simulink model "integrator_12B_with_contracts_Req_TUI003v1_PP"  (R2019b)
settings: Solver=FixedStepDiscrete  StartTime=0.0  StopTime=10.0  FixedStep=1.000000  RelTol=1e-3  EnableMultiTasking=on
model workspace (MAT data in the model file):
  ContractValidatorBlocksMap = containers.Map
  ContractValidatorBlocksMap.serialization.keys = {'integrator_12B/contract/validator', 'integrator_12B_with_contracts/integrator_12B_Tustin_IntegratorSpec/validator', 'integrator_12B_with_contracts_Req_TUI003v1/integrator_12B_Tustin_IntegratorSpec/validator', 'integrator_12B_with_contracts_Req_TUI003v1_PP/integrator_12B_Tustin_IntegratorSpec/validator'}
  ContractValidatorBlocksMap.serialization.values{1}.block = 'integrator_12B/contract/validator'
  ContractValidatorBlocksMap.serialization.values{1}.assumePorts = 0
  ContractValidatorBlocksMap.serialization.values{1}.guaranteePorts = 3
  ContractValidatorBlocksMap.serialization.values{1}.modeBlocksPorts = 0
  ContractValidatorBlocksMap.serialization.values{1}.portHandles.Inport = [741.001708984 742.001708984 743.001708984]
  ContractValidatorBlocksMap.serialization.values{1}.portHandles.Outport = 744.001708984
  ContractValidatorBlocksMap.serialization.values{1}.portHandles.Enable = []
  ContractValidatorBlocksMap.serialization.values{1}.portHandles.Trigger = []
  ContractValidatorBlocksMap.serialization.values{1}.portHandles.State = []
  ContractValidatorBlocksMap.serialization.values{1}.portHandles.LConn = []
  ContractValidatorBlocksMap.serialization.values{1}.portHandles.RConn = []
  ContractValidatorBlocksMap.serialization.values{1}.portHandles.Ifaction = []
  ContractValidatorBlocksMap.serialization.values{1}.portHandles.Reset = []
  ContractValidatorBlocksMap.serialization.values{1}.portConnectivity(1).Type = '1'
  ContractValidatorBlocksMap.serialization.values{1}.portConnectivity(1).Position = [365 -95]
  ContractValidatorBlocksMap.serialization.values{1}.portConnectivity(1).SrcBlock = 540.001953125
  ContractValidatorBlocksMap.serialization.values{1}.portConnectivity(1).SrcPort = 0
  ContractValidatorBlocksMap.serialization.values{1}.portConnectivity(1).DstBlock = []
  ContractValidatorBlocksMap.serialization.values{1}.portConnectivity(1).DstPort = []
  ContractValidatorBlocksMap.serialization.values{1}.portConnectivity(2).Type = '2'
  ContractValidatorBlocksMap.serialization.values{1}.portConnectivity(2).Position = [365 75]
  ContractValidatorBlocksMap.serialization.values{1}.portConnectivity(2).SrcBlock = 544.001953125
  ContractValidatorBlocksMap.serialization.values{1}.portConnectivity(2).SrcPort = 0
  ContractValidatorBlocksMap.serialization.values{1}.portConnectivity(2).DstBlock = []
  ContractValidatorBlocksMap.serialization.values{1}.portConnectivity(2).DstPort = []
  ContractValidatorBlocksMap.serialization.values{1}.portConnectivity(3).Type = '3'
  ContractValidatorBlocksMap.serialization.values{1}.portConnectivity(3).Position = [365 245]
  ContractValidatorBlocksMap.serialization.values{1}.portConnectivity(3).SrcBlock = 548.001953125
  ContractValidatorBlocksMap.serialization.values{1}.portConnectivity(3).SrcPort = 0
  ContractValidatorBlocksMap.serialization.values{1}.portConnectivity(3).DstBlock = []
  ContractValidatorBlocksMap.serialization.values{1}.portConnectivity(3).DstPort = []
  ContractValidatorBlocksMap.serialization.values{1}.portConnectivity(4).Type = '1'
  ContractValidatorBlocksMap.serialization.values{1}.portConnectivity(4).Position = [500 75]
  ContractValidatorBlocksMap.serialization.values{1}.portConnectivity(4).SrcBlock = []
  ContractValidatorBlocksMap.serialization.values{1}.portConnectivity(4).SrcPort = []
  ContractValidatorBlocksMap.serialization.values{1}.portConnectivity(4).DstBlock = 591.001708984
  ContractValidatorBlocksMap.serialization.values{1}.portConnectivity(4).DstPort = 0
  ContractValidatorBlocksMap.serialization.values{2}.block = 'integrator_12B_with_contracts/integrator_12B_Tustin_IntegratorSpec/validator'
  ContractValidatorBlocksMap.serialization.values{2}.assumePorts = 1
  ContractValidatorBlocksMap.serialization.values{2}.guaranteePorts = 1
  ContractValidatorBlocksMap.serialization.values{2}.modeBlocksPorts = 0
  ContractValidatorBlocksMap.serialization.values{2}.portHandles.Inport = [975.177368164 977.177368164]
  ContractValidatorBlocksMap.serialization.values{2}.portHandles.Outport = 1002.17736816
  ContractValidatorBlocksMap.serialization.values{2}.portHandles.Enable = []
  ContractValidatorBlocksMap.serialization.values{2}.portHandles.Trigger = []
  ContractValidatorBlocksMap.serialization.values{2}.portHandles.State = []
  ContractValidatorBlocksMap.serialization.values{2}.portHandles.LConn = []
  ContractValidatorBlocksMap.serialization.values{2}.portHandles.RConn = []
  ContractValidatorBlocksMap.serialization.values{2}.portHandles.Ifaction = []
  ContractValidatorBlocksMap.serialization.values{2}.portHandles.Reset = []
  ContractValidatorBlocksMap.serialization.values{2}.portConnectivity(1).Type = '1'
  ContractValidatorBlocksMap.serialization.values{2}.portConnectivity(1).Position = [1440 910]
  ContractValidatorBlocksMap.serialization.values{2}.portConnectivity(1).SrcBlock = 715.177368164
  ContractValidatorBlocksMap.serialization.values{2}.portConnectivity(1).SrcPort = 0
  ContractValidatorBlocksMap.serialization.values{2}.portConnectivity(1).DstBlock = []
  ContractValidatorBlocksMap.serialization.values{2}.portConnectivity(1).DstPort = []
  ContractValidatorBlocksMap.serialization.values{2}.portConnectivity(2).Type = '2'
  ContractValidatorBlocksMap.serialization.values{2}.portConnectivity(2).Position = [1440 960]
  ContractValidatorBlocksMap.serialization.values{2}.portConnectivity(2).SrcBlock = 723.177368164
  ContractValidatorBlocksMap.serialization.values{2}.portConnectivity(2).SrcPort = 0
  ContractValidatorBlocksMap.serialization.values{2}.portConnectivity(2).DstBlock = []
  ContractValidatorBlocksMap.serialization.values{2}.portConnectivity(2).DstPort = []
  ContractValidatorBlocksMap.serialization.values{2}.portConnectivity(3).Type = '1'
  ContractValidatorBlocksMap.serialization.values{2}.portConnectivity(3).Position = [1480 935]
  ContractValidatorBlocksMap.serialization.values{2}.portConnectivity(3).SrcBlock = []
  ContractValidatorBlocksMap.serialization.values{2}.portConnectivity(3).SrcPort = []
  ContractValidatorBlocksMap.serialization.values{2}.portConnectivity(3).DstBlock = 780.177368164
  ContractValidatorBlocksMap.serialization.values{2}.portConnectivity(3).DstPort = 0
  ContractValidatorBlocksMap.serialization.values{3}.block = 'integrator_12B_with_contracts_Req_TUI003v1/integrator_12B_Tustin_IntegratorSpec/validator'
  ContractValidatorBlocksMap.serialization.values{3}.assumePorts = 1
  ContractValidatorBlocksMap.serialization.values{3}.guaranteePorts = 1
  ContractValidatorBlocksMap.serialization.values{3}.modeBlocksPorts = 0
  ContractValidatorBlocksMap.serialization.values{3}.portHandles.Inport = [223.123657227 224.125366211]
  ContractValidatorBlocksMap.serialization.values{3}.portHandles.Outport = 225.12890625
  ContractValidatorBlocksMap.serialization.values{3}.portHandles.Enable = []
  ContractValidatorBlocksMap.serialization.values{3}.portHandles.Trigger = []
  ContractValidatorBlocksMap.serialization.values{3}.portHandles.State = []
  ContractValidatorBlocksMap.serialization.values{3}.portHandles.LConn = []
  ContractValidatorBlocksMap.serialization.values{3}.portHandles.RConn = []
  ContractValidatorBlocksMap.serialization.values{3}.portHandles.Ifaction = []
  ContractValidatorBlocksMap.serialization.values{3}.portHandles.Reset = []
  ContractValidatorBlocksMap.serialization.values{3}.portConnectivity(1).Type = '1'
  ContractValidatorBlocksMap.serialization.values{3}.portConnectivity(1).Position = [1440 910]
  ContractValidatorBlocksMap.serialization.values{3}.portConnectivity(1).SrcBlock = 127.121582031
  ContractValidatorBlocksMap.serialization.values{3}.portConnectivity(1).SrcPort = 0
  ContractValidatorBlocksMap.serialization.values{3}.portConnectivity(1).DstBlock = []
  ContractValidatorBlocksMap.serialization.values{3}.portConnectivity(1).DstPort = []
  ContractValidatorBlocksMap.serialization.values{3}.portConnectivity(2).Type = '2'
  ContractValidatorBlocksMap.serialization.values{3}.portConnectivity(2).Position = [1440 960]
  ContractValidatorBlocksMap.serialization.values{3}.portConnectivity(2).SrcBlock = 121.124511719
  ContractValidatorBlocksMap.serialization.values{3}.portConnectivity(2).SrcPort = 0
  ContractValidatorBlocksMap.serialization.values{3}.portConnectivity(2).DstBlock = []
  ContractValidatorBlocksMap.serialization.values{3}.portConnectivity(2).DstPort = []
  ContractValidatorBlocksMap.serialization.values{3}.portConnectivity(3).Type = '1'
  ContractValidatorBlocksMap.serialization.values{3}.portConnectivity(3).Position = [1480 935]
  ContractValidatorBlocksMap.serialization.values{3}.portConnectivity(3).SrcBlock = []
  ContractValidatorBlocksMap.serialization.values{3}.portConnectivity(3).SrcPort = []
  ContractValidatorBlocksMap.serialization.values{3}.portConnectivity(3).DstBlock = 149.117919922
  ContractValidatorBlocksMap.serialization.values{3}.portConnectivity(3).DstPort = 0
  ContractValidatorBlocksMap.serialization.values{4}.block = 'integrator_12B_with_contracts_Req_TUI003v1_PP/integrator_12B_Tustin_IntegratorSpec/validator'
  ContractValidatorBlocksMap.serialization.values{4}.assumePorts = 1
  ContractValidatorBlocksMap.serialization.values{4}.guaranteePorts = 1
  ContractValidatorBlocksMap.serialization.values{4}.modeBlocksPorts = 0
  ContractValidatorBlocksMap.serialization.values{4}.portHandles.Inport = [232.125976562 233.154296875]
  ContractValidatorBlocksMap.serialization.values{4}.portHandles.Outport = 234.124511719
  ContractValidatorBlocksMap.serialization.values{4}.portHandles.Enable = []
  ContractValidatorBlocksMap.serialization.values{4}.portHandles.Trigger = []
  ContractValidatorBlocksMap.serialization.values{4}.portHandles.State = []
  ContractValidatorBlocksMap.serialization.values{4}.portHandles.LConn = []
  ContractValidatorBlocksMap.serialization.values{4}.portHandles.RConn = []
  ContractValidatorBlocksMap.serialization.values{4}.portHandles.Ifaction = []
  ContractValidatorBlocksMap.serialization.values{4}.portHandles.Reset = []
  ContractValidatorBlocksMap.serialization.values{4}.portConnectivity(1).Type = '1'
  ContractValidatorBlocksMap.serialization.values{4}.portConnectivity(1).Position = [1440 910]
  ContractValidatorBlocksMap.serialization.values{4}.portConnectivity(1).SrcBlock = 127.121704102
  ContractValidatorBlocksMap.serialization.values{4}.portConnectivity(1).SrcPort = 0
  ContractValidatorBlocksMap.serialization.values{4}.portConnectivity(1).DstBlock = []
  ContractValidatorBlocksMap.serialization.values{4}.portConnectivity(1).DstPort = []
  ContractValidatorBlocksMap.serialization.values{4}.portConnectivity(2).Type = '2'
  ContractValidatorBlocksMap.serialization.values{4}.portConnectivity(2).Position = [1440 960]
  ContractValidatorBlocksMap.serialization.values{4}.portConnectivity(2).SrcBlock = 121.124633789
  ContractValidatorBlocksMap.serialization.values{4}.portConnectivity(2).SrcPort = 0
  ContractValidatorBlocksMap.serialization.values{4}.portConnectivity(2).DstBlock = []
  ContractValidatorBlocksMap.serialization.values{4}.portConnectivity(2).DstPort = []
  ContractValidatorBlocksMap.serialization.values{4}.portConnectivity(3).Type = '1'
  ContractValidatorBlocksMap.serialization.values{4}.portConnectivity(3).Position = [1480 935]
  ContractValidatorBlocksMap.serialization.values{4}.portConnectivity(3).SrcBlock = []
  ContractValidatorBlocksMap.serialization.values{4}.portConnectivity(3).SrcPort = []
  ContractValidatorBlocksMap.serialization.values{4}.portConnectivity(3).DstBlock = 158.119506836
  ContractValidatorBlocksMap.serialization.values{4}.portConnectivity(3).DstPort = 0
  ContractValidatorBlocksMap.serialization.uniformity = 0
  ContractValidatorBlocksMap.serialization.keyType = 'char'
  ContractValidatorBlocksMap.serialization.valueType = 'any'
  already_pp = 1
  compositionalMap.analysisNames{1} = 'integrator_12B_with_contracts_Req_TUI003v1_PP/Tustin
    | Integrator
    | (Limited, Resettable, States)'
  compositionalMap.compositionalOptions = {{''}}
  compositionalMap.selectedOptions = 1
  maskControlsMap = containers.Map
  maskControlsMap.serialization.keys = {'integrator_12B_with_contracts_Req_TUI003v1_PP/integrator_12B_Tustin_IntegratorSpec/TUI003v1'}
  maskControlsMap.serialization.values = {{'Display_counter_example_as_signals', 'Display_counter_example_as_tables', 'Display_counter_example_as_HTML_tables', 'Generate_an_outer_model_for_the_counter_example', 'Generate_an_inner_model_for_the_counter_example'}}
  maskControlsMap.serialization.uniformity = 0
  maskControlsMap.serialization.keyType = 'char'
  maskControlsMap.serialization.valueType = 'any'
  nodeNameToBlockNameMap = containers.Map
  nodeNameToBlockNameMap.serialization.keys = {'A_1', 'A_equal__equal__gt_B_1', 'Arrow_xxTustin_IntegratorSpec_7_ni_1_1', 'BL_1', 'BLc_1', 'B_1', 'Gain_1', 'In1_1', 'Logical_newline_Operator1_1', 'Logical_newline_Operator_1', 'LowerRelop1_1', 'PRE_xxTustin_IntegratorSpec_11_1', 'PRE_xxTustin_IntegratorSpec_9_1', 'Product_1', 'RelationalOperator_1', 'Saturation_newline_Dynamic_1', 'Saturation_newline_Dynamic_22_119', 'Sum1_1', 'Sum_1', 'Switch1_1', 'Switch2_1', 'Switch_1', 'TL_1', 'TLc_1', 'TUI003v1_1', 'TUI003v1_121_125', 'T_1', 'Tustin_IntegratorSpec_BL_1', 'Tustin_IntegratorSpec_IC_1', 'Tustin_IntegratorSpec_RESET_1', 'Tustin_IntegratorSpec_TL_1', 'Tustin_IntegratorSpec_T_1', 'Tustin_IntegratorSpec_xin_1', 'Tustin_IntegratorSpec_yout_1', 'Tustin_newline_Integrator_newline__lpar_Limited_comma_Resettable_comma_States_rpar__1', 'Tustin_newline_Integrator_newline__lpar_Limited_comma_Resettable_comma_States_rpar__9_120', 'UnitDelay1_1', 'UnitDelay_1', 'UpperRelop_1', 'assume_1', 'assume_127_122', 'bounds_1', 'bounds_2', 'bounds_63_125', 'branch_8_IF_1', 'branch_9_IF_1', 'guarantee_1', 'ic_1', 'integrator_12B_Tustin_IntegratorSpec_110_125', 'integrator_12B_with_contracts_Req_TUI003v1_PP', 'lo_1', 'normal_yout_operator_1', 'normalv1_operator_1', 'reset_1', 'spec137_operator_1', 'spec160_operator_1', 'spec160_operator_136_119', 'u_1', 'up_1', 'valid_1', 'xin_1', 'xxTustin_IntegratorSpec_13_operator_1', 'xxTustin_IntegratorSpec_14_operator_1', 'xxTustin_IntegratorSpec_15_operator_1', 'xxTustin_IntegratorSpec_16_operator_1', 'xxTustin_IntegratorSpec_1_operator_1', 'xxTustin_IntegratorSpec_4_operator_1', 'xxTustin_IntegratorSpec_5_operator_1', 'xxTustin_IntegratorSpec_5_rhs_2_1', 'xxTustin_IntegratorSpec_6_operator_1', 'xxTustin_IntegratorSpec_7_ni_1_init_1', 'xxTustin_IntegratorSpec_8_rhs_1', 'y_1', 'yout_1'}
  nodeNameToBlockNameMap.serialization.values{1} = 'integrator_12B_with_contracts_Req_TUI003v1_PP/integrator_12B_Tustin_IntegratorSpec/spec160_operator/A'
  nodeNameToBlockNameMap.serialization.values{2} = 'integrator_12B_with_contracts_Req_TUI003v1_PP/integrator_12B_Tustin_IntegratorSpec/spec160_operator/A ==> B'
  nodeNameToBlockNameMap.serialization.values{3} = 'integrator_12B_with_contracts_Req_TUI003v1_PP/integrator_12B_Tustin_IntegratorSpec/Arrow_xxTustin_IntegratorSpec_7_ni_1'
  nodeNameToBlockNameMap.serialization.values{4} = 'integrator_12B_with_contracts_Req_TUI003v1_PP/BL'
  nodeNameToBlockNameMap.serialization.values{5} = 'integrator_12B_with_contracts_Req_TUI003v1_PP/Tustin
    | Integrator
    | (Limited, Resettable, States)/bounds/BLc'
  nodeNameToBlockNameMap.serialization.values{6} = 'integrator_12B_with_contracts_Req_TUI003v1_PP/integrator_12B_Tustin_IntegratorSpec/spec160_operator/B'
  nodeNameToBlockNameMap.serialization.values{7} = 'integrator_12B_with_contracts_Req_TUI003v1_PP/Tustin
    | Integrator
    | (Limited, Resettable, States)/Gain'
  nodeNameToBlockNameMap.serialization.values{8} = 'integrator_12B_with_contracts_Req_TUI003v1_PP/integrator_12B_Tustin_IntegratorSpec/assume/In1'
  nodeNameToBlockNameMap.serialization.values{9} = 'integrator_12B_with_contracts_Req_TUI003v1_PP/integrator_12B_Tustin_IntegratorSpec/spec160_operator/Logical
    | Operator1'
  nodeNameToBlockNameMap.serialization.values{10} = 'integrator_12B_with_contracts_Req_TUI003v1_PP/integrator_12B_Tustin_IntegratorSpec/spec160_operator/Logical
    | Operator'
  nodeNameToBlockNameMap.serialization.values{11} = 'integrator_12B_with_contracts_Req_TUI003v1_PP/Tustin
    | Integrator
    | (Limited, Resettable, States)/Saturation
    | Dynamic/LowerRelop1'
  nodeNameToBlockNameMap.serialization.values{12} = 'integrator_12B_with_contracts_Req_TUI003v1_PP/integrator_12B_Tustin_IntegratorSpec/PRE_xxTustin_IntegratorSpec_11'
  nodeNameToBlockNameMap.serialization.values{13} = 'integrator_12B_with_contracts_Req_TUI003v1_PP/integrator_12B_Tustin_IntegratorSpec/PRE_xxTustin_IntegratorSpec_9'
  nodeNameToBlockNameMap.serialization.values{14} = 'integrator_12B_with_contracts_Req_TUI003v1_PP/Tustin
    | Integrator
    | (Limited, Resettable, States)/Product'
  nodeNameToBlockNameMap.serialization.values{15} = 'integrator_12B_with_contracts_Req_TUI003v1_PP/Tustin
    | Integrator
    | (Limited, Resettable, States)/bounds/Relational Operator'
  nodeNameToBlockNameMap.serialization.values{16} = 'integrator_12B_with_contracts_Req_TUI003v1_PP/Tustin
    | Integrator
    | (Limited, Resettable, States)/Saturation
    | Dynamic'
  nodeNameToBlockNameMap.serialization.values{17} = 'integrator_12B_with_contracts_Req_TUI003v1_PP/Tustin
    | Integrator
    | (Limited, Resettable, States)/Saturation
    | Dynamic'
  nodeNameToBlockNameMap.serialization.values{18} = 'integrator_12B_with_contracts_Req_TUI003v1_PP/Tustin
    | Integrator
    | (Limited, Resettable, States)/Sum1'
  nodeNameToBlockNameMap.serialization.values{19} = 'integrator_12B_with_contracts_Req_TUI003v1_PP/Tustin
    | Integrator
    | (Limited, Resettable, States)/Sum'
  nodeNameToBlockNameMap.serialization.values{20} = 'integrator_12B_with_contracts_Req_TUI003v1_PP/Tustin
    | Integrator
    | (Limited, Resettable, States)/bounds/Switch1'
  nodeNameToBlockNameMap.serialization.values{21} = 'integrator_12B_with_contracts_Req_TUI003v1_PP/Tustin
    | Integrator
    | (Limited, Resettable, States)/bounds/Switch2'
  nodeNameToBlockNameMap.serialization.values{22} = 'integrator_12B_with_contracts_Req_TUI003v1_PP/Tustin
    | Integrator
    | (Limited, Resettable, States)/Switch'
  nodeNameToBlockNameMap.serialization.values{23} = 'integrator_12B_with_contracts_Req_TUI003v1_PP/TL'
  nodeNameToBlockNameMap.serialization.values{24} = 'integrator_12B_with_contracts_Req_TUI003v1_PP/Tustin
    | Integrator
    | (Limited, Resettable, States)/bounds/TLc'
  nodeNameToBlockNameMap.serialization.values{25} = 'integrator_12B_with_contracts_Req_TUI003v1_PP/integrator_12B_Tustin_IntegratorSpec/TUI003v1'
  nodeNameToBlockNameMap.serialization.values{26} = 'integrator_12B_with_contracts_Req_TUI003v1_PP/integrator_12B_Tustin_IntegratorSpec/TUI003v1'
  nodeNameToBlockNameMap.serialization.values{27} = 'integrator_12B_with_contracts_Req_TUI003v1_PP/T'
  nodeNameToBlockNameMap.serialization.values{28} = 'integrator_12B_with_contracts_Req_TUI003v1_PP/integrator_12B_Tustin_IntegratorSpec/Tustin_IntegratorSpec_BL'
  nodeNameToBlockNameMap.serialization.values{29} = 'integrator_12B_with_contracts_Req_TUI003v1_PP/integrator_12B_Tustin_IntegratorSpec/Tustin_IntegratorSpec_IC'
  nodeNameToBlockNameMap.serialization.values{30} = 'integrator_12B_with_contracts_Req_TUI003v1_PP/integrator_12B_Tustin_IntegratorSpec/Tustin_IntegratorSpec_RESET'
  nodeNameToBlockNameMap.serialization.values{31} = 'integrator_12B_with_contracts_Req_TUI003v1_PP/integrator_12B_Tustin_IntegratorSpec/Tustin_IntegratorSpec_TL'
  nodeNameToBlockNameMap.serialization.values{32} = 'integrator_12B_with_contracts_Req_TUI003v1_PP/integrator_12B_Tustin_IntegratorSpec/Tustin_IntegratorSpec_T'
  nodeNameToBlockNameMap.serialization.values{33} = 'integrator_12B_with_contracts_Req_TUI003v1_PP/integrator_12B_Tustin_IntegratorSpec/Tustin_IntegratorSpec_xin'
  nodeNameToBlockNameMap.serialization.values{34} = 'integrator_12B_with_contracts_Req_TUI003v1_PP/integrator_12B_Tustin_IntegratorSpec/Tustin_IntegratorSpec_yout'
  nodeNameToBlockNameMap.serialization.values{35} = 'integrator_12B_with_contracts_Req_TUI003v1_PP/Tustin
    | Integrator
    | (Limited, Resettable, States)'
  nodeNameToBlockNameMap.serialization.values{36} = 'integrator_12B_with_contracts_Req_TUI003v1_PP/Tustin
    | Integrator
    | (Limited, Resettable, States)'
  nodeNameToBlockNameMap.serialization.values{37} = 'integrator_12B_with_contracts_Req_TUI003v1_PP/Tustin
    | Integrator
    | (Limited, Resettable, States)/Unit Delay1'
  nodeNameToBlockNameMap.serialization.values{38} = 'integrator_12B_with_contracts_Req_TUI003v1_PP/Tustin
    | Integrator
    | (Limited, Resettable, States)/Unit Delay'
  nodeNameToBlockNameMap.serialization.values{39} = 'integrator_12B_with_contracts_Req_TUI003v1_PP/Tustin
    | Integrator
    | (Limited, Resettable, States)/Saturation
    | Dynamic/UpperRelop'
  nodeNameToBlockNameMap.serialization.values{40} = 'integrator_12B_with_contracts_Req_TUI003v1_PP/integrator_12B_Tustin_IntegratorSpec/assume'
  nodeNameToBlockNameMap.serialization.values{41} = 'integrator_12B_with_contracts_Req_TUI003v1_PP/integrator_12B_Tustin_IntegratorSpec/assume'
  nodeNameToBlockNameMap.serialization.values{42} = 'integrator_12B_with_contracts_Req_TUI003v1_PP/Tustin
    | Integrator
    | (Limited, Resettable, States)/bounds'
  nodeNameToBlockNameMap.serialization.values{43} = 'integrator_12B_with_contracts_Req_TUI003v1_PP/Tustin
    | Integrator
    | (Limited, Resettable, States)/bounds'
  nodeNameToBlockNameMap.serialization.values{44} = 'integrator_12B_with_contracts_Req_TUI003v1_PP/Tustin
    | Integrator
    | (Limited, Resettable, States)/bounds'
  nodeNameToBlockNameMap.serialization.values{45} = 'integrator_12B_with_contracts_Req_TUI003v1_PP/integrator_12B_Tustin_IntegratorSpec/branch_8_IF'
  nodeNameToBlockNameMap.serialization.values{46} = 'integrator_12B_with_contracts_Req_TUI003v1_PP/integrator_12B_Tustin_IntegratorSpec/branch_9_IF'
  nodeNameToBlockNameMap.serialization.values{47} = 'integrator_12B_with_contracts_Req_TUI003v1_PP/integrator_12B_Tustin_IntegratorSpec/TUI003v1/guarantee'
  nodeNameToBlockNameMap.serialization.values{48} = 'integrator_12B_with_contracts_Req_TUI003v1_PP/ic'
  nodeNameToBlockNameMap.serialization.values{49} = 'integrator_12B_with_contracts_Req_TUI003v1_PP/integrator_12B_Tustin_IntegratorSpec/assume'
  nodeNameToBlockNameMap.serialization.values{50} = 'integrator_12B_with_contracts_Req_TUI003v1_PP'
  nodeNameToBlockNameMap.serialization.values{51} = 'integrator_12B_with_contracts_Req_TUI003v1_PP/Tustin
    | Integrator
    | (Limited, Resettable, States)/Saturation
    | Dynamic/lo'
  nodeNameToBlockNameMap.serialization.values{52} = 'integrator_12B_with_contracts_Req_TUI003v1_PP/integrator_12B_Tustin_IntegratorSpec/normal_yout_operator'
  nodeNameToBlockNameMap.serialization.values{53} = 'integrator_12B_with_contracts_Req_TUI003v1_PP/integrator_12B_Tustin_IntegratorSpec/normalv1_operator'
  nodeNameToBlockNameMap.serialization.values{54} = 'integrator_12B_with_contracts_Req_TUI003v1_PP/reset'
  nodeNameToBlockNameMap.serialization.values{55} = 'integrator_12B_with_contracts_Req_TUI003v1_PP/integrator_12B_Tustin_IntegratorSpec/spec137_operator'
  nodeNameToBlockNameMap.serialization.values{56} = 'integrator_12B_with_contracts_Req_TUI003v1_PP/integrator_12B_Tustin_IntegratorSpec/spec160_operator'
  nodeNameToBlockNameMap.serialization.values{57} = 'integrator_12B_with_contracts_Req_TUI003v1_PP/integrator_12B_Tustin_IntegratorSpec/spec160_operator'
  nodeNameToBlockNameMap.serialization.values{58} = 'integrator_12B_with_contracts_Req_TUI003v1_PP/Tustin
    | Integrator
    | (Limited, Resettable, States)/Saturation
    | Dynamic/u'
  nodeNameToBlockNameMap.serialization.values{59} = 'integrator_12B_with_contracts_Req_TUI003v1_PP/Tustin
    | Integrator
    | (Limited, Resettable, States)/Saturation
    | Dynamic/up'
  nodeNameToBlockNameMap.serialization.values{60} = 'integrator_12B_with_contracts_Req_TUI003v1_PP/integrator_12B_Tustin_IntegratorSpec/valid'
  nodeNameToBlockNameMap.serialization.values{61} = 'integrator_12B_with_contracts_Req_TUI003v1_PP/xin'
  nodeNameToBlockNameMap.serialization.values{62} = 'integrator_12B_with_contracts_Req_TUI003v1_PP/integrator_12B_Tustin_IntegratorSpec/xxTustin_IntegratorSpec_13_operator'
  nodeNameToBlockNameMap.serialization.values{63} = 'integrator_12B_with_contracts_Req_TUI003v1_PP/integrator_12B_Tustin_IntegratorSpec/xxTustin_IntegratorSpec_14_operator'
  nodeNameToBlockNameMap.serialization.values{64} = 'integrator_12B_with_contracts_Req_TUI003v1_PP/integrator_12B_Tustin_IntegratorSpec/xxTustin_IntegratorSpec_15_operator'
  nodeNameToBlockNameMap.serialization.values{65} = 'integrator_12B_with_contracts_Req_TUI003v1_PP/integrator_12B_Tustin_IntegratorSpec/xxTustin_IntegratorSpec_16_operator'
  nodeNameToBlockNameMap.serialization.values{66} = 'integrator_12B_with_contracts_Req_TUI003v1_PP/integrator_12B_Tustin_IntegratorSpec/xxTustin_IntegratorSpec_1_operator'
  nodeNameToBlockNameMap.serialization.values{67} = 'integrator_12B_with_contracts_Req_TUI003v1_PP/integrator_12B_Tustin_IntegratorSpec/xxTustin_IntegratorSpec_4_operator'
  nodeNameToBlockNameMap.serialization.values{68} = 'integrator_12B_with_contracts_Req_TUI003v1_PP/integrator_12B_Tustin_IntegratorSpec/xxTustin_IntegratorSpec_5_operator'
  nodeNameToBlockNameMap.serialization.values{69} = 'integrator_12B_with_contracts_Req_TUI003v1_PP/integrator_12B_Tustin_IntegratorSpec/xxTustin_IntegratorSpec_5_rhs_2'
  nodeNameToBlockNameMap.serialization.values{70} = 'integrator_12B_with_contracts_Req_TUI003v1_PP/integrator_12B_Tustin_IntegratorSpec/xxTustin_IntegratorSpec_6_operator'
  nodeNameToBlockNameMap.serialization.values{71} = 'integrator_12B_with_contracts_Req_TUI003v1_PP/integrator_12B_Tustin_IntegratorSpec/xxTustin_IntegratorSpec_7_ni_1_init'
  nodeNameToBlockNameMap.serialization.values{72} = 'integrator_12B_with_contracts_Req_TUI003v1_PP/integrator_12B_Tustin_IntegratorSpec/xxTustin_IntegratorSpec_8_rhs'
  nodeNameToBlockNameMap.serialization.values{73} = 'integrator_12B_with_contracts_Req_TUI003v1_PP/Tustin
    | Integrator
    | (Limited, Resettable, States)/Saturation
    | Dynamic/y'
  nodeNameToBlockNameMap.serialization.values{74} = 'integrator_12B_with_contracts_Req_TUI003v1_PP/yout'
  nodeNameToBlockNameMap.serialization.uniformity = 1
  nodeNameToBlockNameMap.serialization.keyType = 'char'
  nodeNameToBlockNameMap.serialization.valueType = 'char'
  verificationResults : object (value not decoded)
undefined symbols (not defined in the file): contractAfterSimulation, ContractAssumeBlock, contractBeforeSimulation, ContractBlock, ContractGuaranteeBlock, ContractValidatorBlock, saveValidatorParameters
settings Model: Creator=elliocm  LastModifiedBy=hbourbou
settings DataIOCC: LimitDataPoints=on  SaveFormat=Array  ReturnWorkspaceOutputs=off
settings OptimizationCC: ExpressionDepthLimit=2147483647  LifeSpan=inf
settings DebuggingCC: AlgebraicLoopMsg=error  ArtificialAlgebraicLoopMsg=error  UnderspecifiedInitializationDetection=Classic  MergeDetectMultiDrivingBlocksExec=none  SolverPrmCheckMsg=warning  SingleTaskRateTransMsg=error  IntegerOverflowMsg=none  StateNameClashWarn=warning  SFUnexpectedBacktrackingDiag=warning  SFNoUnconditionalDefaultTransitionDiag=warning  SFExecutionAtInitializationDiag=none  IntegerSaturationMsg=none  ArithmeticOperatorsInVariantConditions=warning
settings HardwareCC: ProdBitPerPointer=32  ProdBitPerSizeT=32  ProdBitPerPtrDiffT=32  ProdLargestAtomicFloat=None  ProdIntDivRoundTo=Undefined  ProdEndianess=Unspecified  ProdWordSize=32  ProdHWDeviceType=32-bit Generic
settings ModelReferenceCC: PropagateSignalLabelsOutOfModel=off
settings SFSimCC: SimUseLocalCustomCode=off  CustomCodeUndefinedFunction=UseInterfaceOnly
settings RTWCC: RTWUseLocalCustomCode=off
settings CodeAppCC: StateflowObjectComments=on
settings GRTTargetCC: TargetLangStandard=C89/C90 (ANSI)  GeneratePreprocessorConditionals=Disable all
settings ConfigComp: CovMetricSettings=dw  CovHtmlReporting=on  CovSaveCumulativeToWorkspaceVar=on  CovSaveSingleToWorkspaceVar=on  CovExternalEMLEnable=off  DVMaxProcessTime=5000  DVMaxTestCaseSteps=500  DVTestSuiteOptimization=CombinedObjectives (Nonlinear Extended)  DVDetectActiveLogic=on

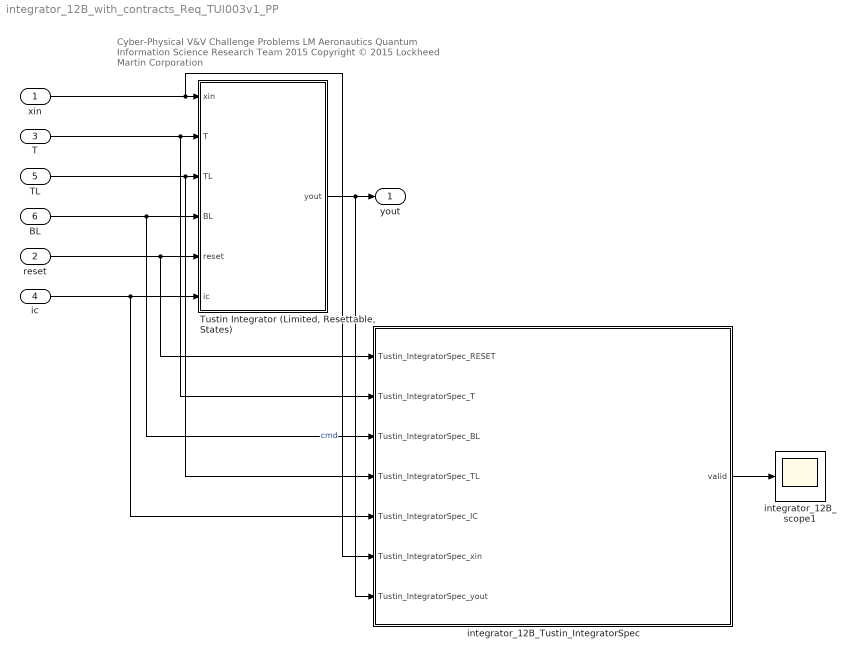
== system integrator_12B_with_contracts_Req_TUI003v1_PP ==
  note: Cyber-Physical V&V Challenge Problems
      | LM Aeronautics Quantum Information Science Research Team 2015
      | Copyright © 2015 Lockheed Martin Corporation
  xin : Inport  OutDataTypeStr=double
  reset : Inport  Port=2  OutDataTypeStr=boolean
  T : Inport  Port=3  OutDataTypeStr=double
  ic : Inport  Port=4  OutDataTypeStr=double
  TL : Inport  Port=5  OutDataTypeStr=double
  BL : Inport  Port=6  OutDataTypeStr=double
  "Tustin Integrator (Limited, Resettable, States)" : Subsystem  TreatAsAtomicUnit=on
  integrator_12B_Tustin_IntegratorSpec : Subsystem  TreatAsAtomicUnit=on  mask(ContractBlock){ContractBlockType=ContractBlock}
      mask init:
      | set_param(gcb, 'LinkStatus', 'none');
      mask DialogControl DescTextVar Prompt: Contract block
      mask Display:
      | text(0.5, 0.5, '{\bf\fontsize{20}Contract}', 'hor', 'center', 'texmode','on');
      | blocks = find_system(gcb, 'LookUnderMasks','all', 'SearchDepth',1,'BlockType','Inport');
      | for i = 1 : length(blocks)
      |     blockName = get_param(blocks(i), 'Name');
      |     [path, blockName] = fileparts(char(blockName));
      |     port_label('input', i, blockName);
      | end
      | 
      | blocks = find_system(gcb, 'LookUnderMasks','all', 'SearchDepth',1,'BlockType','Outport');
      | for i = 1 : length(blocks)
      |     blockName = get_param(blocks(i), 'Name');
      |     [path, blockName] = fileparts(char(blockName));
      |     port_label('output', i, blockName);
      | end
  integrator_12B_scope1 : Scope
  yout : Outport  VectorParamsAs1DForOutWhenUnconnected=off
  wires:
  BL/1 -> integrator_12B_Tustin_IntegratorSpec/3(Tustin_IntegratorSpec_BL), "Tustin Integrator (Limited, Resettable, States)"/4(BL)
  TL/1 -> "Tustin Integrator (Limited, Resettable, States)"/3(TL), integrator_12B_Tustin_IntegratorSpec/4(Tustin_IntegratorSpec_TL)
  reset/1 -> integrator_12B_Tustin_IntegratorSpec/1(Tustin_IntegratorSpec_RESET), "Tustin Integrator (Limited, Resettable, States)"/5(reset)
  ic/1 -> integrator_12B_Tustin_IntegratorSpec/5(Tustin_IntegratorSpec_IC), "Tustin Integrator (Limited, Resettable, States)"/6(ic)
  "Tustin Integrator (Limited, Resettable, States)"/1(yout) -> yout/1, integrator_12B_Tustin_IntegratorSpec/7(Tustin_IntegratorSpec_yout)
  T/1 -> "Tustin Integrator (Limited, Resettable, States)"/2(T), integrator_12B_Tustin_IntegratorSpec/2(Tustin_IntegratorSpec_T)
  xin/1 -> "Tustin Integrator (Limited, Resettable, States)"/1(xin), integrator_12B_Tustin_IntegratorSpec/6(Tustin_IntegratorSpec_xin)  "cmd"
  integrator_12B_Tustin_IntegratorSpec/1(valid) -> integrator_12B_scope1/1

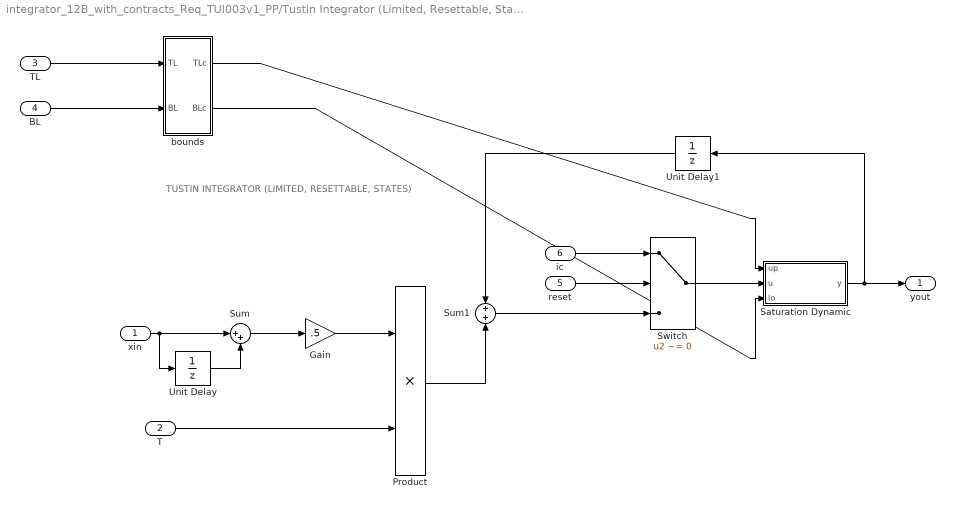
== system integrator_12B_with_contracts_Req_TUI003v1_PP/Tustin Integrator (Limited, Resettable, States) ==
  note: TUSTIN INTEGRATOR (LIMITED, RESETTABLE, STATES)
  xin : Inport
  T : Inport  Port=2
  TL : Inport  Port=3
  BL : Inport  Port=4
  reset : Inport  Port=5
  ic : Inport  Port=6
  Gain : Gain  Gain=.5
  Product : Product  RndMeth=Zero
  Saturation Dynamic : Subsystem  TreatAsAtomicUnit=on  mask(Saturation Dynamic){OutMin=[], OutMax=[], OutDataTypeStr=Inherit: Same as second input, OutputDataTypeScalingMode=Same as second input, OutDataType=fixdt(1, 16), OutScaling=2^-10, LockScale=off, RndMeth=Floor, DoSatur=off}
      mask prompts: OutMin "Simulink:masks:OutputMinimum_MP"; OutMax "Simulink:masks:OutputMaximum_MP"; OutDataTypeStr "Simulink:masks:OutputDataType_MP"; OutputDataTypeScalingMode "Simulink:masks:OutputDataTypeMode_MP"; OutDataType "Simulink:masks:OutputDataTypeegFixdt116Fixdtsingle_MP"; OutScaling "Simulink:masks:OutputScalingSlopeEg29OrSlopeBias_MP"; LockScale "Simulink:masks:LockOutputDataTypeAgainstFxpTools_MP"; RndMeth "Simulink:masks:IntegerRoundingMode_MP"; DoSatur "Simulink:masks:SaturateOnIntegerOverflow_MP"
      mask help: Simulink:masks:SaturationDynamic_MD
      mask init:
      | blkH = gcbh;
      | blkName = getfullname(blkH);
      | 
      | switch_blks = {'Switch','Switch2'}; 
      | for i = 1:length(switch_blks)
      |   set_param([blkName,'/',switch_blks{i}], ...
      |       'RndMeth', RndMeth, ...
      | 	  'DoSatur', DoSatur);
      | end
      | 
      | propBlk = [blkName, '/Data Type Propagation'];
      | 
      | if strcmp(OutputDataTypeScalingMode, 'Same as second input')
      |     set_param(propBlk, 'PropDataTypeMode', 'Inherit via propagation rule', ...
      |                        'PropScalingMode',  'Inherit via propagation rule');
      | else
      |     scaling = OutScaling;
      |     scalingMode = 'Specify via dialog';
      |     switch OutputDataTypeScalingMode
      |       case 'double'
      |         dataType = 'fixdt(''double'')';
      |       case 'single'
      |         dataType = 'fixdt(''single'')';
      |       case 'int8'
      |         dataType = 'fixdt(1,8,0)';
      |       case 'uint8'
      |         dataType = 'fixdt(0,8,0)';
      |       case 'int16'
      |         dataType = 'fixdt(1,16,0)';
      |       case 'uint16'
      |         dataType = 'fixdt(0,16,0)';
      |       case 'int32'
      |         dataType = 'fixdt(1,32,0)';
      |       case 'uint32'
      |         dataType = 'fixdt(0,32,0)';
      |       case 'Specify via dialog'
      |         dataType = OutDataType;
      |         if ~isempty(OutDataTypeStr) && isa(OutDataTypeStr,'Simulink.NumericType') 
      |           if strcmp(OutDataTypeStr.DataTypeMode, 'Fixed-point: unspecified scaling') 
      |             scalingMode = 'Obtain via best precision';
      |             range = [OutMin OutMax];
      |             range = range(~isinf(range));
      |             set_param(propBlk, 'ValuesUsedBestPrec', mat2str(range));
      |           end
      |         end
      |     end
      |     
      |     set_param(propBlk, 'PropDataTypeMode', 'Specify via dialog', ...
      |                        'PropScalingMode',  scalingMode, ...
      |                        'PropDataType',     dataType, ...
      |                        'PropScaling',      scaling);
      | end
      mask Callback OutDataTypeStr: fixptdialog(gcbh)
      mask TypeOptions OutputDataTypeScalingMode: double | single | int8 | uint8 | int16 | uint16 | int32 | uint32 | Specify via dialog | Same as second input
      mask Callback OutputDataTypeScalingMode: fixptdialog(gcbh)
      mask Callback OutDataType: fixptdialog(gcbh)
      mask TypeOptions RndMeth: Simulink:masks:Ceiling | Simulink:masks:Convergent | Simulink:masks:Floor | Simulink:masks:Nearest | Simulink:masks:Round | Simulink:masks:Simplest | Simulink:masks:Zero
  Sum : Sum  Inputs=|++
  Sum1 : Sum
  Switch : Switch  Criteria=u2 ~= 0  Threshold=0.5
  Unit Delay : UnitDelay  SampleTime=-1  HasFrameUpgradeWarning=on
  Unit Delay1 : UnitDelay  SampleTime=-1  HasFrameUpgradeWarning=on
  bounds : Subsystem  TreatAsAtomicUnit=on
  yout : Outport  VectorParamsAs1DForOutWhenUnconnected=off
  wires:
  xin/1 -> Unit Delay/1, Sum/1
  Unit Delay/1 -> Sum/2
  Sum/1 -> Gain/1
  Gain/1 -> Product/1
  T/1 -> Product/2
  Product/1 -> Sum1/2
  Sum1/1 -> Switch/3
  reset/1 -> Switch/2
  ic/1 -> Switch/1
  Switch/1 -> Saturation Dynamic/2(u)
  Saturation Dynamic/1(y) -> Unit Delay1/1, yout/1
  Unit Delay1/1 -> Sum1/1
  TL/1 -> bounds/1(TL)
  BL/1 -> bounds/2(BL)
  bounds/1(TLc) -> Saturation Dynamic/1(up)
  bounds/2(BLc) -> Saturation Dynamic/3(lo)

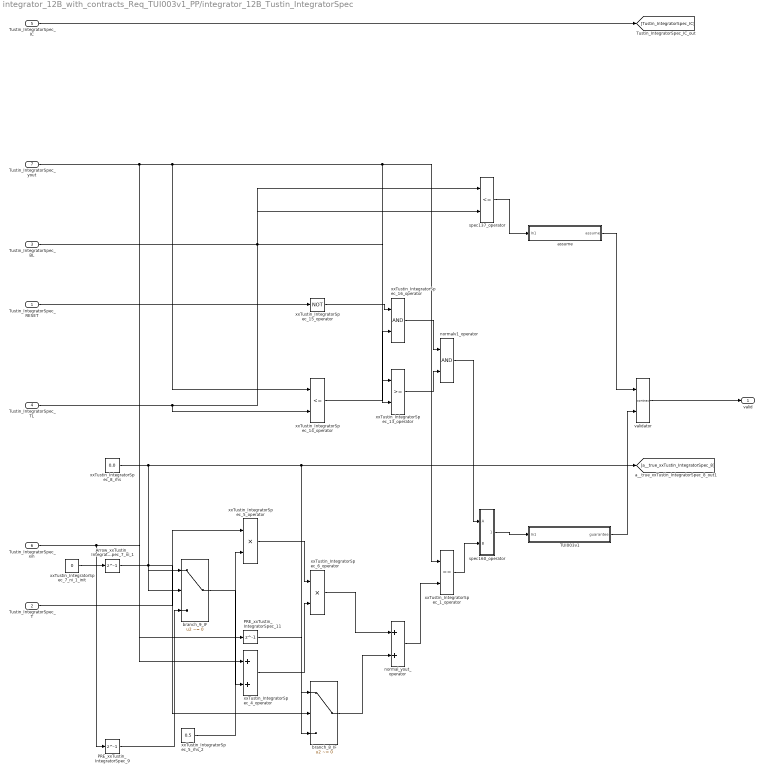
== system integrator_12B_with_contracts_Req_TUI003v1_PP/integrator_12B_Tustin_IntegratorSpec ==
  Tustin_IntegratorSpec_RESET : Inport  OutDataTypeStr=boolean
  Tustin_IntegratorSpec_T : Inport  Port=2  OutDataTypeStr=double
  Tustin_IntegratorSpec_BL : Inport  Port=3  OutDataTypeStr=double
  Tustin_IntegratorSpec_TL : Inport  Port=4  OutDataTypeStr=double
  Tustin_IntegratorSpec_IC : Inport  Port=5  OutDataTypeStr=double
  Tustin_IntegratorSpec_xin : Inport  Port=6  OutDataTypeStr=double
  Tustin_IntegratorSpec_yout : Inport  Port=7  OutDataTypeStr=double
  Arrow_xxTustin_IntegratorSpec_7_ni_1 : Delay  DelayLength=1  InitialCondition=1
  PRE_xxTustin_IntegratorSpec_11 : Delay  DelayLength=1  InitialCondition=0
  PRE_xxTustin_IntegratorSpec_9 : Delay  DelayLength=1  InitialCondition=0
  TUI003v1 : Subsystem  TreatAsAtomicUnit=on  mask(ContractGuaranteeBlock){ContractBlockType=ContractGuaranteeBlock}
      mask init:
      | set_param(gcb, 'LinkStatus', 'none');
      mask DialogControl DescTextVar Prompt: Guarantee block
      mask DialogControl Display_counter_example_as_signals Prompt: Display counter example as signals
      mask DialogControl Display_counter_example_as_signals Callback: displayCexSignals(1, 1);
      mask DialogControl Display_counter_example_as_tables Prompt: Display counter example as tables
      mask DialogControl Display_counter_example_as_tables Callback: displayCexTables(1, 1);
      mask DialogControl Display_counter_example_as_HTML_tables Prompt: Display counter example as HTML tables
      mask DialogControl Display_counter_example_as_HTML_tables Callback: displayCexHtmlTables(1, 1);
      mask DialogControl Generate_an_outer_model_for_the_counter_example Prompt: Generate an outer model for the counter example
      mask DialogControl Generate_an_outer_model_for_the_counter_example Callback: generateModelWithSignalBuilders(1, 1, 2);
      mask DialogControl Generate_an_inner_model_for_the_counter_example Prompt: Generate an inner model for the counter example
      mask DialogControl Generate_an_inner_model_for_the_counter_example Callback: generateModelWithSignalBuilders(1, 1, 1);
  assume : Subsystem  TreatAsAtomicUnit=on  mask(ContractAssumeBlock){ContractBlockType=ContractAssumeBlock}
      mask init:
      | set_param(gcb, 'LinkStatus', 'none');
      mask DialogControl DescTextVar Prompt: Assume block
  branch_8_IF : Switch  Criteria=u2 ~= 0
  branch_9_IF : Switch  Criteria=u2 ~= 0
  normal_yout_operator : Sum  OutDataTypeStr=double
  normalv1_operator : Logic  AllPortsSameDT=off  OutDataTypeStr=boolean
  spec137_operator : RelationalOperator  Operator=<=  OutDataTypeStr=boolean  RndMeth=Simplest
  spec160_operator : Subsystem  TreatAsAtomicUnit=on
  validator : M-S-Function  LoadFcn=saveValidatorParameters(gcb);  InitFcn=contractBeforeSimulation();  StopFcn=contractAfterSimulation();  FunctionName=contract  mask(ContractValidatorBlock){assumePorts=1, guaranteePorts=1, modePorts=0, ContractBlockType=ContractValidatorBlock, createInportsCheckbox=off}
      mask prompts: assumePorts "Assume ports     :"; guaranteePorts "Guarantee ports :"; modePorts "Mode ports        :"; createInportsCheckbox "Create inports and connect them automatically"
      mask init:
      | set_param(gcb,'LinkStatus','none');
      | contract_callback('inputs_callback',gcb);
      mask DialogControl DescTextVar Prompt: The validator block implements the following logic: <br> <br> <b>Sofar</b>(assume<sub>1</sub> <b>&#8743;</b> assume<sub>2</sub> <b>&#8743;</b> ... assume<sub>k</sub>) <b>&rarr;</b> (guarantee<sub>1</sub> <b>&#8743;</b> guarantee<sub>2</sub> <b>&#8743;</b> ... guarantee<sub>m</sub> <b>&#8743;</b>  mode<sub>1</sub> <b>&#8743;</b> mode<sub>2</sub> <b>&#8743;</b> ... <b>&#8743;</b> mode<sub>n</sub> )<br> where mode<sub>i</sub> = require<sub>i</sub> <b>&rarr;</b> ensure<sub>i</sub>
      mask Display:
      | color('black');
      | port_label('input',1,'assume');
      | port_label('input',2,'guarantee');
      | port_label('output',1,'valid');
  xxTustin_IntegratorSpec_13_operator : RelationalOperator  OutDataTypeStr=boolean  RndMeth=Simplest
  xxTustin_IntegratorSpec_14_operator : RelationalOperator  Operator=<=  OutDataTypeStr=boolean  RndMeth=Simplest
  xxTustin_IntegratorSpec_15_operator : Logic  Operator=NOT  AllPortsSameDT=off  OutDataTypeStr=boolean
  xxTustin_IntegratorSpec_16_operator : Logic  AllPortsSameDT=off  OutDataTypeStr=boolean
  xxTustin_IntegratorSpec_1_operator : RelationalOperator  Operator===  OutDataTypeStr=boolean  RndMeth=Simplest
  xxTustin_IntegratorSpec_4_operator : Sum  OutDataTypeStr=double
  xxTustin_IntegratorSpec_5_operator : Product  OutDataTypeStr=double
  xxTustin_IntegratorSpec_5_rhs_2 : Constant  Value=0.5  OutDataTypeStr=double
  xxTustin_IntegratorSpec_6_operator : Product  OutDataTypeStr=double
  xxTustin_IntegratorSpec_7_ni_1_init : Constant  Value=0  OutDataTypeStr=boolean
  xxTustin_IntegratorSpec_8_rhs : Constant  Value=0.0  OutDataTypeStr=double
  valid : Outport
  wires:
  validator/1 -> valid/1
  xxTustin_IntegratorSpec_4_operator/1 -> xxTustin_IntegratorSpec_6_operator/2
  xxTustin_IntegratorSpec_5_operator/1 -> xxTustin_IntegratorSpec_6_operator/1
  xxTustin_IntegratorSpec_5_rhs_2/1 -> xxTustin_IntegratorSpec_5_operator/2
  Tustin_IntegratorSpec_T/1 -> xxTustin_IntegratorSpec_5_operator/1
  branch_9_IF/1 -> xxTustin_IntegratorSpec_4_operator/2
  normal_yout_operator/1 -> xxTustin_IntegratorSpec_1_operator/2
  xxTustin_IntegratorSpec_14_operator/1 -> xxTustin_IntegratorSpec_16_operator/2
  xxTustin_IntegratorSpec_15_operator/1 -> xxTustin_IntegratorSpec_16_operator/1
  Tustin_IntegratorSpec_RESET/1 -> xxTustin_IntegratorSpec_15_operator/1
  TUI003v1/1(guarantee) -> validator/2
  assume/1(assume) -> validator/1
  xxTustin_IntegratorSpec_1_operator/1 -> spec160_operator/2(B)
  normalv1_operator/1 -> spec160_operator/1(A)
  xxTustin_IntegratorSpec_13_operator/1 -> normalv1_operator/2
  xxTustin_IntegratorSpec_16_operator/1 -> normalv1_operator/1
  branch_8_IF/1 -> normal_yout_operator/2
  xxTustin_IntegratorSpec_6_operator/1 -> normal_yout_operator/1
  spec160_operator/1(A ==> B) -> TUI003v1/1(In1)
  PRE_xxTustin_IntegratorSpec_9/1 -> branch_9_IF/3
  PRE_xxTustin_IntegratorSpec_11/1 -> branch_8_IF/3
  spec137_operator/1 -> assume/1(In1)
  Tustin_IntegratorSpec_IC/1 -> [Tustin_IntegratorSpec_IC]
  xxTustin_IntegratorSpec_7_ni_1_init/1 -> Arrow_xxTustin_IntegratorSpec_7_ni_1/1
  Tustin_IntegratorSpec_yout/1 -> xxTustin_IntegratorSpec_1_operator/1, xxTustin_IntegratorSpec_13_operator/1, xxTustin_IntegratorSpec_14_operator/1, PRE_xxTustin_IntegratorSpec_11/1
  Tustin_IntegratorSpec_TL/1 -> xxTustin_IntegratorSpec_14_operator/2, spec137_operator/2
  Tustin_IntegratorSpec_BL/1 -> xxTustin_IntegratorSpec_13_operator/2, spec137_operator/1
  Tustin_IntegratorSpec_xin/1 -> xxTustin_IntegratorSpec_4_operator/1, PRE_xxTustin_IntegratorSpec_9/1
  xxTustin_IntegratorSpec_8_rhs/1 -> branch_8_IF/1, [a__true_xxTustin_IntegratorSpec_8], branch_9_IF/1
  Arrow_xxTustin_IntegratorSpec_7_ni_1/1 -> branch_9_IF/2, branch_8_IF/2

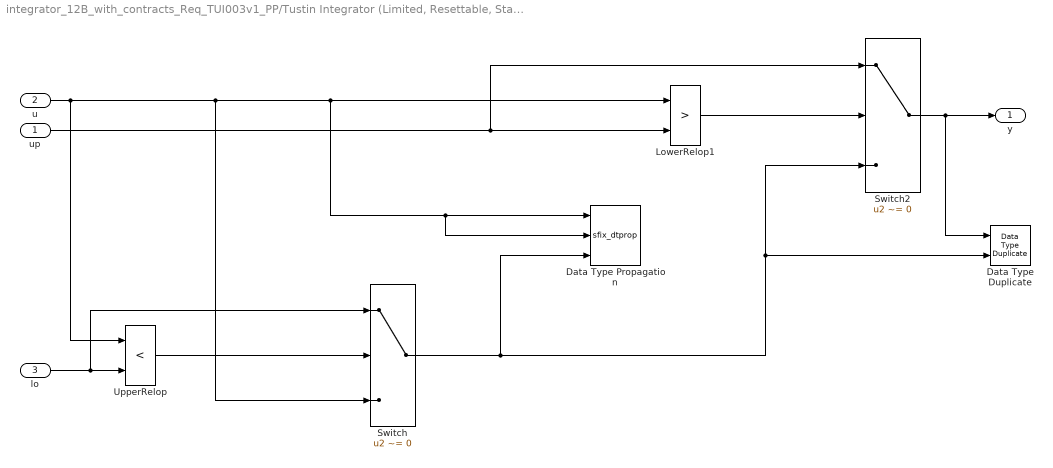
== system integrator_12B_with_contracts_Req_TUI003v1_PP/Tustin Integrator (Limited, Resettable, States)/Saturation Dynamic ==
  up : Inport
  u : Inport  Port=2
  lo : Inport  Port=3
  Data Type Duplicate : DataTypeDuplicate  DisableCoverage=on
  Data Type Propagation : S-Function  FunctionName=sfix_dtprop  Parameters=14,PropDataTypeMode,(getdatatypespecs(PropDataType,PropScaling,DblOver,0, 0, PropDataTypeMode, PropScalingMode)),IfRefDouble,IfRefSingle,IsSigned,NumBitsBase,NumBitsMult,NumBitsAdd,(sort(reshape(round(NumBitsAllowFinal), prod(size(NumBitsAllowFinal)),1))),PropScalingMode,ValuesUsedBestPrec,SlopeBase,SlopeMult,SlopeAdd,BiasBase,BiasMult,BiasAdd,DblOver  SFunctionDeploymentMode=off  EnableBusSupport=off  mask(Data Type Propagation){PropDataTypeMode=Inherit via propagation rule, PropDataType=fixdt(1, 16), IfRefDouble=double, IfRefSingle=single, IsSigned=IsSigned1, NumBitsBase=NumBits1, NumBitsMult=1, NumBitsAdd=0, NumBitsAllowFinal=1:128, PropScalingMode=Inherit via propagation rule, PropScaling=2^-10, ValuesUsedBestPrec=[5 -7], SlopeBase=Slope1, SlopeMult=1, SlopeAdd=0, BiasBase=Bias1, BiasMult=1, BiasAdd=0}
      mask prompts: PropDataTypeMode "Simulink:masks:x1PropagatedDataType_MP"; PropDataType "Simulink:masks:x11PropagatedDataTypeegFixdt116Fixdtsingle_MP"; IfRefDouble "Simulink:masks:x11IfAnyReferenceInputIsDoubleOutputIs_MP"; IfRefSingle "Simulink:masks:x12IfAnyReferenceInputIsSingleOutputIs_MP"; IsSigned "Simulink:masks:x13IsSigned_MP"; NumBitsBase "Simulink:masks:x141NumberofBitsBase_MP"; NumBitsMult "Simulink:masks:x142NumberofBitsMultiplicativeAdjustment_MP"; NumBitsAdd "Simulink:masks:x143NumberofBitsAdditiveAdjustment_MP"; NumBitsAllowFinal "Simulink:masks:x144NumberofBitsAllowableFinalValues_MP"; PropScalingMode "Simulink:masks:x2PropagatedScaling_MP"; PropScaling "Simulink:masks:x21PropagatedScalingSlopeEg29OrSlopeBiasEg1253_MP"; ValuesUsedBestPrec "Simulink:masks:x21ValuesUsedToDetermineBestPrecisionScaling_MP"; SlopeBase "Simulink:masks:x211SlopeBase_MP"; SlopeMult "Simulink:masks:x212SlopeMultiplicativeAdjustment_MP"; SlopeAdd "Simulink:masks:x213SlopeAdditiveAdjustment_MP"; BiasBase "Simulink:masks:x221BiasBase_MP"; BiasMult "Simulink:masks:x222BiasMultiplicativeAdjustment_MP"; BiasAdd "Simulink:masks:x223BiasAdditiveAdjustment_MP"
      mask help: Simulink:masks:DataTypePropagation_MD
      mask init:
      | DblOver = 0;
      mask TypeOptions PropDataTypeMode: Simulink:masks:SpecifyViaDialog | Simulink:masks:InheritViaPropagationRule
      mask Callback PropDataTypeMode: fixptdialog(gcbh)
      mask Callback PropDataType: fixptdialog(gcbh)
      mask TypeOptions IfRefDouble: Simulink:masks:double | Simulink:masks:single
      mask TypeOptions IfRefSingle: Simulink:masks:double | Simulink:masks:single
      mask TypeOptions IsSigned: Simulink:masks:IsSigned1 | Simulink:masks:IsSigned2 | Simulink:masks:IsSigned1OrIsSigned2 | Simulink:masks:TRUE | Simulink:masks:FALSE
      mask TypeOptions NumBitsBase: NumBits1 | NumBits2 | max([NumBits1 NumBits2]) | min([NumBits1 NumBits2]) | NumBits1+NumBits2
      mask TypeOptions PropScalingMode: Simulink:masks:SpecifyViaDialog | Simulink:masks:InheritViaPropagationRule | Simulink:masks:ObtainViaBestPrecision
      mask Callback PropScalingMode: fixptdialog(gcbh)
      mask TypeOptions SlopeBase: Slope1 | Slope2 | max([Slope1 Slope2]) | min([Slope1 Slope2]) | Slope1*Slope2 | Slope1/Slope2 | PosRange1 | PosRange2 | max([PosRange1 PosRange2]) | min([PosRange1 PosRange2]) | PosRange1*PosRange2 | PosRange1/PosRange2
      mask TypeOptions BiasBase: Bias1 | Bias2 | max([Bias1 Bias2]) | min([Bias1 Bias2]) | Bias1*Bias2 | Bias1/Bias2 | Bias1+Bias2 | Bias1-Bias2
      mask Display:
      | port_label('Input',1,'Ref1');
      | port_label('Input',2,'Ref2');
      | port_label('Input',3,'Prop');
  LowerRelop1 : RelationalOperator  DisableCoverage=on  Operator=>  OutDataTypeStr=boolean  RndMeth=Nearest
  Switch : Switch  Criteria=u2 ~= 0  OutDataTypeStr=Inherit: Inherit via back propagation  ZeroCross=off
  Switch2 : Switch  Criteria=u2 ~= 0  OutMin=OutMin  OutMax=OutMax  OutDataTypeStr=Inherit: Inherit via back propagation  ZeroCross=off
  UpperRelop : RelationalOperator  DisableCoverage=on  Operator=<  OutDataTypeStr=boolean  RndMeth=Nearest
  y : Outport  OutMin=OutMin  OutMax=OutMax  VectorParamsAs1DForOutWhenUnconnected=off
  wires:
  up/1 -> Switch2/1, LowerRelop1/2
  u/1 -> Data Type Propagation/2, Data Type Propagation/1, LowerRelop1/1, Switch/3, UpperRelop/1
  lo/1 -> Switch/1, UpperRelop/2
  Switch/1 -> Data Type Duplicate/2, Switch2/3, Data Type Propagation/3
  Switch2/1 -> Data Type Duplicate/1, y/1
  LowerRelop1/1 -> Switch2/2
  UpperRelop/1 -> Switch/2

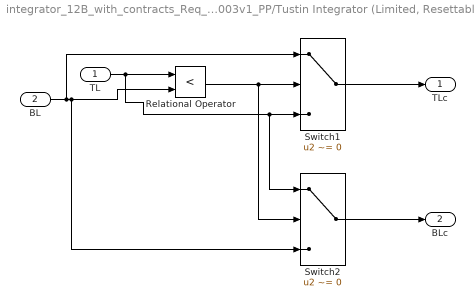
== system integrator_12B_with_contracts_Req_TUI003v1_PP/Tustin Integrator (Limited, Resettable, States)/bounds ==
  TL : Inport
  BL : Inport  Port=2
  Relational Operator : RelationalOperator  Operator=<  OutDataTypeStr=boolean  RndMeth=Nearest
  Switch1 : Switch  Criteria=u2 ~= 0  Threshold=0.5
  Switch2 : Switch  Criteria=u2 ~= 0  Threshold=0.5
  TLc : Outport  VectorParamsAs1DForOutWhenUnconnected=off
  BLc : Outport  Port=2  VectorParamsAs1DForOutWhenUnconnected=off
  wires:
  BL/1 -> Switch1/1, Switch2/3, Relational Operator/2
  TL/1 -> Switch2/1, Switch1/3, Relational Operator/1
  Relational Operator/1 -> Switch2/2, Switch1/2
  Switch1/1 -> TLc/1
  Switch2/1 -> BLc/1

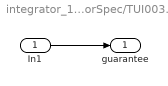
== system integrator_12B_with_contracts_Req_TUI003v1_PP/integrator_12B_Tustin_IntegratorSpec/TUI003v1 ==
  In1 : Inport
  guarantee : Outport  OutDataTypeStr=boolean
  wires:
  In1/1 -> guarantee/1

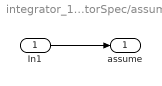
== system integrator_12B_with_contracts_Req_TUI003v1_PP/integrator_12B_Tustin_IntegratorSpec/assume ==
  In1 : Inport
  assume : Outport  OutDataTypeStr=boolean
  wires:
  In1/1 -> assume/1

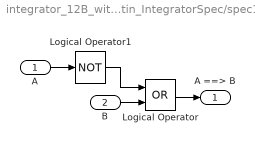
== system integrator_12B_with_contracts_Req_TUI003v1_PP/integrator_12B_Tustin_IntegratorSpec/spec160_operator ==
  A : Inport
  B : Inport  Port=2
  Logical Operator : Logic  Operator=OR  AllPortsSameDT=off  OutDataTypeStr=boolean
  Logical Operator1 : Logic  Operator=NOT  AllPortsSameDT=off  OutDataTypeStr=boolean
  A ==> B : Outport  VectorParamsAs1DForOutWhenUnconnected=off
  wires:
  B/1 -> Logical Operator/2
  A/1 -> Logical Operator1/1
  Logical Operator/1 -> A ==> B/1
  Logical Operator1/1 -> Logical Operator/1
